simulink model "regulator_LQR_discrete_comparison"  (R2021b)
settings: Solver=ode45  StartTime=0.0  StopTime=tsim  RelTol=1e-3  EnableMultiTasking=on
values from neighbouring files (symbols this model uses):
  C_states = eye(2)    [es_4.m]
  D_states = [0 0]'    [es_4.m]
  KdlqrSat = Kdlqr    [es_4.m]
  sat_max = umax    (= 5)    [es_4.m]
  sat_min = umin    (= -5)    [es_4.m]
  sysd = c2d(sys,Ts)    [es_4.m]
  Ts = 0.1    [es_4.m]
  x0 = [0 10]'    [es_4.m]
  xref = [0 0]'    [es_4.m]
undefined symbols (not defined in the file or in its folder): Kdlqr, KdlqrSat2
settings Model: Creator=Administrator  LastModifiedBy=PaoloA
settings SolverCC: AlgebraicLoopSolver=TrustRegion
settings DataIOCC: LimitDataPoints=on  SaveFormat=Array  SignalLoggingSaveFormat=ModelDataLogs  ReturnWorkspaceOutputs=off
settings OptimizationCC: ExpressionDepthLimit=2147483647  InitFltsAndDblsToZero=on  LifeSpan=inf
settings DebuggingCC: UnderspecifiedInitializationDetection=Classic  MergeDetectMultiDrivingBlocksExec=none  SolverPrmCheckMsg=warning  FcnCallInpInsideContextMsg=warning  StateNameClashWarn=warning  SFUnexpectedBacktrackingDiag=warning  SFNoUnconditionalDefaultTransitionDiag=warning  SFExecutionAtInitializationDiag=none  SFMachineParentedDataDiag=warning  ArithmeticOperatorsInVariantConditions=warning
settings HardwareCC: ProdBitPerPointer=32  ProdBitPerSizeT=32  ProdBitPerPtrDiffT=32  ProdLargestAtomicFloat=None  ProdIntDivRoundTo=Undefined  ProdEndianess=Unspecified  ProdWordSize=32  ProdHWDeviceType=32-bit Generic
settings ModelReferenceCC: PropagateSignalLabelsOutOfModel=off
settings SFSimCC: SimUseLocalCustomCode=off  CustomCodeUndefinedFunction=UseInterfaceOnly
settings RTWCC: RTWUseLocalCustomCode=off
settings CodeAppCC: StateflowObjectComments=on
settings GRTTargetCC: TargetLangStandard=C89/C90 (ANSI)  CombineOutputUpdateFcns=off  GRTInterface=on
settings ConfigComp: CovMetricSettings=dw  CovSaveCumulativeToWorkspaceVar=on  CovSaveSingleToWorkspaceVar=on  CovExternalEMLEnable=off  CovSFcnEnable=off

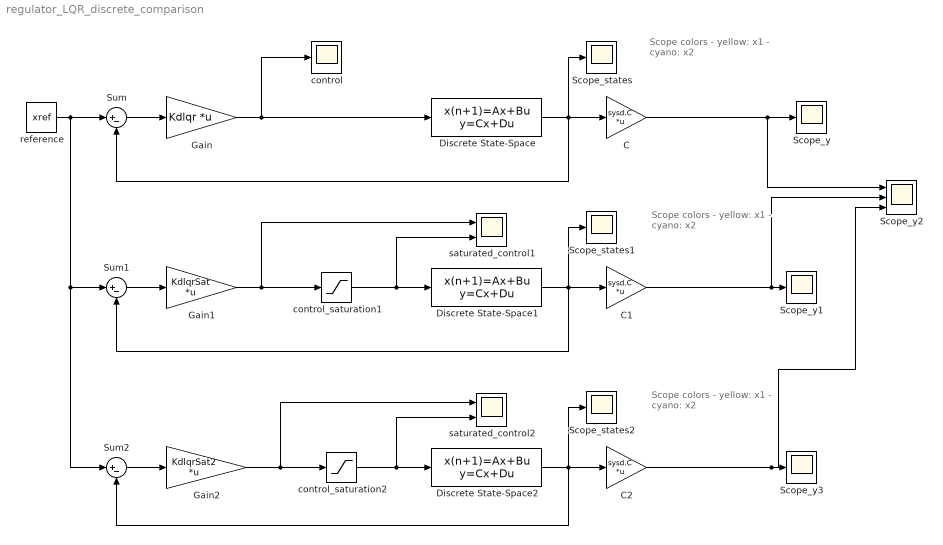
== system regulator_LQR_discrete_comparison ==
  note: Scope colors
      | - yellow: x1
      | - cyano: x2
  note: Scope colors
      | - yellow: x1
      | - cyano: x2
  note: Scope colors
      | - yellow: x1
      | - cyano: x2
  C : Gain  Gain=sysd.C  Multiplication=Matrix(K*u)
  C1 : Gain  Gain=sysd.C  Multiplication=Matrix(K*u)
  C2 : Gain  Gain=sysd.C  Multiplication=Matrix(K*u)
  Discrete State-Space : DiscreteStateSpace  A=sysd.A  B=sysd.B  C=C_states  D=D_states  InitialCondition=x0  SampleTime=Ts
  Discrete State-Space1 : DiscreteStateSpace  A=sysd.A  B=sysd.B  C=C_states  D=D_states  InitialCondition=x0  SampleTime=Ts
  Discrete State-Space2 : DiscreteStateSpace  A=sysd.A  B=sysd.B  C=C_states  D=D_states  InitialCondition=x0  SampleTime=Ts
  Gain : Gain  Gain=Kdlqr  Multiplication=Matrix(K*u)
  Gain1 : Gain  Gain=KdlqrSat  Multiplication=Matrix(K*u)
  Gain2 : Gain  Gain=KdlqrSat2  Multiplication=Matrix(K*u)
  Scope_states : Scope
  Scope_states1 : Scope
  Scope_states2 : Scope
  Scope_y : Scope
  Scope_y1 : Scope
  Scope_y2 : Scope  NumInputPorts=3
  Scope_y3 : Scope
  Sum : Sum  Inputs=|+-
  Sum1 : Sum  Inputs=|+-
  Sum2 : Sum  Inputs=|+-
  control : Scope
  control_saturation1 : Saturate  UpperLimit=sat_max  LowerLimit=sat_min
  control_saturation2 : Saturate  UpperLimit=sat_max  LowerLimit=sat_min
  reference : Constant  Value=xref
  saturated_control1 : Scope  NumInputPorts=2
  saturated_control2 : Scope  NumInputPorts=2
  wires:
  Gain/1 -> Discrete State-Space/1, control/1
  Sum/1 -> Gain/1
  Discrete State-Space/1 -> C/1, Scope_states/1, Sum/2
  C/1 -> Scope_y2/1, Scope_y/1
  C1/1 -> Scope_y2/2, Scope_y1/1
  Discrete State-Space1/1 -> C1/1, Scope_states1/1, Sum1/2
  Gain1/1 -> saturated_control1/1, control_saturation1/1
  control_saturation1/1 -> Discrete State-Space1/1, saturated_control1/2
  Sum1/1 -> Gain1/1
  Discrete State-Space2/1 -> C2/1, Scope_states2/1, Sum2/2
  Sum2/1 -> Gain2/1
  reference/1 -> Sum2/1, Sum1/1, Sum/1
  control_saturation2/1 -> Discrete State-Space2/1, saturated_control2/2
  Gain2/1 -> saturated_control2/1, control_saturation2/1
  C2/1 -> Scope_y2/3, Scope_y3/1
